simulink model "SwarmSMC1"  (R2022a)
settings: Solver=FixedStepAuto  StartTime=0.0  StopTime=50  FixedStep=0.001  RelTol=1e-3
libraries: slpidlib x26
(part 1 of 3)
settings Model: SimulationMode=rapid-accelerator  Creator=贺嘉辣  LastModifiedBy=YYL
settings SolverCC: AlgebraicLoopSolver=TrustRegion
settings DebuggingCC: UnconnectedInputMsg=warning  UnconnectedOutputMsg=warning  UnconnectedLineMsg=warning  SFMachineParentedDataDiag=warning
settings RTWCC: DLArmComputeVersion=19.05

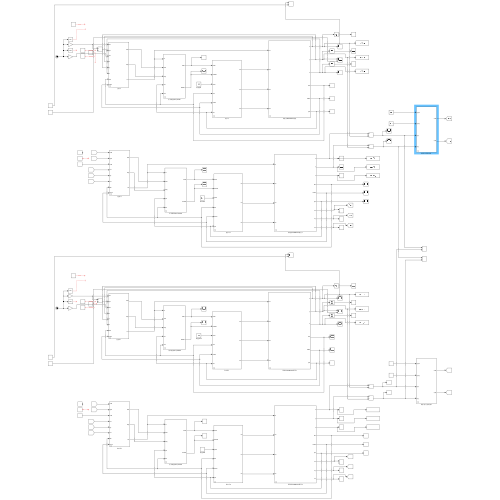
[thumbnail: Simulink's stored preview of the top-level diagram]
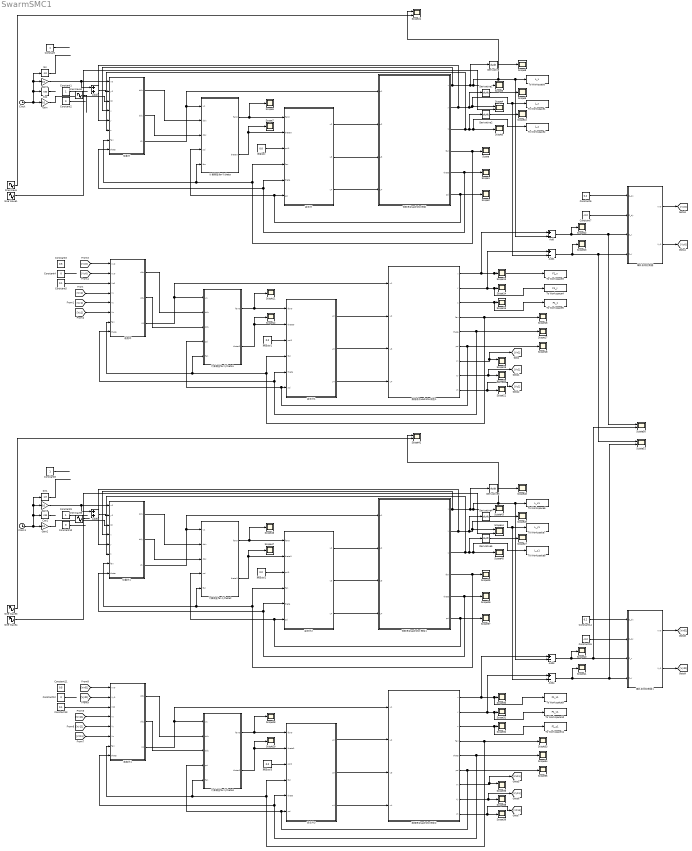
== system SwarmSMC1 ==
  Add{,1,3..4} (4 alike) : Sum  Inputs=+-
  Add2 : Sum
  Add5 : Sum
  Clock : Clock
  Clock1 : Clock
  Constant{,1,8..9} (4 alike) : Constant
  Constant{2,4,10,12} (4 alike) : Constant  Value=0
  Constant11 : Constant  Value=0.5
  Constant13 : Constant  Value=0.1
  Constant14 : Constant  Value=0.2
  Constant15 : Constant  Value=-0.2
  Constant3 : Constant  Value=0.5
  Constant5 : Constant  Value=0.1
  Constant6 : Constant  Value=0.2
  Constant7 : Constant  Value=-0.2
  Cos : Trigonometry  Operator=cos
  Cos1 : Trigonometry  Operator=cos
  Derivative{,1..5} (6 alike) : Derivative
  Gain{,1..3} (4 alike) : Gain  Gain=0.1
  Scope{,1..3,5..18,20..23,25..35,37..41,43,45..49} (44 alike) : Scope
  Scope{4,19,24,36,42,44,50..51} (8 alike) : Scope  NumInputPorts=2
  Sin : Trigonometry
  Sin1 : Trigonometry
  Sine Wave : Sin  Frequency=0.2  SampleTime=0
  Sine Wave1 : Sin  Frequency=0.2  Phase=pi/2  SampleTime=0
  Sine Wave2 : Sin  Amplitude=2.5  Frequency=0.04  SampleTime=0
  Sine Wave3 : Sin  Frequency=0.2  SampleTime=0
  Sine Wave4 : Sin  Frequency=0.2  Phase=pi/2  SampleTime=0
  Sine Wave5 : Sin  Amplitude=2.5  Frequency=0.04  SampleTime=0
  To Workspace : ToWorkspace  VariableName=L_x  SaveFormat=Timeseries  SampleTime=-1
  To Workspace1 : ToWorkspace  VariableName=L_y  SaveFormat=Timeseries  SampleTime=-1
  To Workspace10 : ToWorkspace  VariableName=F1_y1  SaveFormat=Timeseries  SampleTime=-1
  To Workspace11 : ToWorkspace  VariableName=F1_z1  SaveFormat=Timeseries  SampleTime=-1
  To Workspace2 : ToWorkspace  VariableName=L_z  SaveFormat=Timeseries  SampleTime=-1
  To Workspace3 : ToWorkspace  VariableName=F1_x  SaveFormat=Timeseries  SampleTime=-1
  To Workspace4 : ToWorkspace  VariableName=F1_y  SaveFormat=Timeseries  SampleTime=-1
  To Workspace5 : ToWorkspace  VariableName=F1_z  SaveFormat=Timeseries  SampleTime=-1
  To Workspace6 : ToWorkspace  VariableName=L_x1  SaveFormat=Timeseries  SampleTime=-1
  To Workspace7 : ToWorkspace  VariableName=L_y1  SaveFormat=Timeseries  SampleTime=-1
  To Workspace8 : ToWorkspace  VariableName=L_z1  SaveFormat=Timeseries  SampleTime=-1
  To Workspace9 : ToWorkspace  VariableName=F1_x1  SaveFormat=Timeseries  SampleTime=-1
  位置环 : Subsystem  mask{m=0.65, g=9.8}
      mask prompts: m "无人机质量"; g "重力加速度"
  位置环1 : Subsystem  mask{m=0.65, g=9.8}
      mask prompts: m "无人机质量"; g "重力加速度"
  姿态环 : Subsystem  mask{Ixx=7.5e-3, Iyy=7.5e-3, Izz=1.3e-2}
      mask prompts: Ixx "无人机绕X轴转动惯量"; Iyy "无人机绕Y轴转动惯量"; Izz "无人机绕Z轴转动惯量"
  姿态环1 : Subsystem  mask{Ixx=7.5e-3, Iyy=7.5e-3, Izz=1.3e-2}
      mask prompts: Ixx "无人机绕X轴转动惯量"; Iyy "无人机绕Y轴转动惯量"; Izz "无人机绕Z轴转动惯量"
  姿态环2 : Subsystem  mask{Ixx=7.5e-3, Iyy=7.5e-3, Izz=1.3e-2}
      mask prompts: Ixx "无人机绕X轴转动惯量"; Iyy "无人机绕Y轴转动惯量"; Izz "无人机绕Z轴转动惯量"
  姿态环3 : Subsystem  mask{Ixx=7.5e-3, Iyy=7.5e-3, Izz=1.3e-2}
      mask prompts: Ixx "无人机绕X轴转动惯量"; Iyy "无人机绕Y轴转动惯量"; Izz "无人机绕Z轴转动惯量"
  期望psi{,1..3} (4 alike) : Constant  Value=0.0
  编队协同控制器 : Subsystem  mask{m=0.65, g=9.8}
      mask prompts: m "无人机质量"; g "重力加速度"
  编队协同控制器1 : Subsystem  mask{m=0.65, g=9.8}
      mask prompts: m "无人机质量"; g "重力加速度"
  计算期望fan与theta : Subsystem  mask{m=0.65}
      mask prompts: m "无人机质量"
  计算期望fan与theta1 : Subsystem  mask{m=0.65}
      mask prompts: m "无人机质量"
  计算期望fan与theta2 : Subsystem  mask{m=0.65}
      mask prompts: m "无人机质量"
  计算期望fan与theta3 : Subsystem  mask{m=0.65}
      mask prompts: m "无人机质量"
  跟随者Quadrotor模型1 : Subsystem  mask{m=0.65, g=9.8, Ixx=7.5e-3, Iyy=7.5e-3, Izz=1.3e-2, L=0.23, rho=3.1e-5, gama=7.5e-7}
      mask prompts: m "无人机质量"; g "重力加速度"; Ixx "四旋翼绕X轴转动惯量"; Iyy "四旋翼绕Y轴转动惯量"; Izz "四旋翼绕Z轴转动惯量"; L "四旋翼臂长"; rho "四旋翼升力系数"; gama "空气阻力系数"
  跟随者Quadrotor模型2 : Subsystem  mask{m=0.65, g=9.8, Ixx=7.5e-3, Iyy=7.5e-3, Izz=1.3e-2, L=0.23, rho=3.1e-5, gama=7.5e-7}
      mask prompts: m "无人机质量"; g "重力加速度"; Ixx "四旋翼绕X轴转动惯量"; Iyy "四旋翼绕Y轴转动惯量"; Izz "四旋翼绕Z轴转动惯量"; L "四旋翼臂长"; rho "四旋翼升力系数"; gama "空气阻力系数"
  速度环 : Subsystem  mask{m=0.65, g=9.8}
      mask prompts: m "无人机质量"; g "重力加速度"
  速度环1 : Subsystem  mask{m=0.65, g=9.8}
      mask prompts: m "无人机质量"; g "重力加速度"
  领航者Quadrotor模型 : Subsystem  mask{m=0.65, g=9.8, Ixx=7.5e-3, Iyy=7.5e-3, Izz=1.3e-2, L=0.23, rho=3.1e-5, gama=7.5e-7}
      mask prompts: m "无人机质量"; g "重力加速度"; Ixx "四旋翼绕X轴转动惯量"; Iyy "四旋翼绕Y轴转动惯量"; Izz "四旋翼绕Z轴转动惯量"; L "四旋翼臂长"; rho "四旋翼升力系数"; gama "空气阻力系数"
  领航者Quadrotor模型1 : Subsystem  mask{m=0.65, g=9.8, Ixx=7.5e-3, Iyy=7.5e-3, Izz=1.3e-2, L=0.23, rho=3.1e-5, gama=7.5e-7}
      mask prompts: m "无人机质量"; g "重力加速度"; Ixx "四旋翼绕X轴转动惯量"; Iyy "四旋翼绕Y轴转动惯量"; Izz "四旋翼绕Z轴转动惯量"; L "四旋翼臂长"; rho "四旋翼升力系数"; gama "空气阻力系数"
  wires:
  姿态环/3(u4) -> 领航者Quadrotor模型/4(u4)
  姿态环/2(u3) -> 领航者Quadrotor模型/3(u3)
  姿态环/1(u2) -> 领航者Quadrotor模型/2(u2)
  领航者Quadrotor模型/5(theta) -> Scope1/1, 位置环/8(theta), 姿态环/5(theta)
  领航者Quadrotor模型/6(psi) -> Scope2/1, 计算期望fan与theta/4(psi), 姿态环/6(psi)
  领航者Quadrotor模型/4(fan) -> Scope/1, 姿态环/4(fan), 位置环/7(fan), 计算期望fan与theta/5(fan)
  领航者Quadrotor模型/1(x) -> 位置环/4(x), Derivative/1, Scope24/1, Add/2, To Workspace/1, Scope3/1
  领航者Quadrotor模型/2(y) -> 位置环/5(y), Derivative1/1, Scope4/1, Add1/2, To Workspace1/1
  领航者Quadrotor模型/3(z) -> 位置环/6(z), Derivative2/1, To Workspace2/1, Scope5/1
  期望psi/1 -> 姿态环/3(psi0)
  计算期望fan与theta/2(theta0) -> Scope7/1, 姿态环/2(theta0)
  计算期望fan与theta/1(fan0) -> 姿态环/1(fan0), Scope6/1
  位置环/1(ddx) -> 计算期望fan与theta/2(ddx)
  位置环/2(ddy) -> 计算期望fan与theta/3(ddy)
  位置环/3(U1) -> 领航者Quadrotor模型/1(u1), 计算期望fan与theta/1(u1)
  Clock/1 -> Gain/1, Gain1/1, Sin/1, Cos/1
  Constant/1 -> ?
  Constant1/1 -> ?
  Constant2/1 -> ?
  Derivative/1 -> Scope8/1
  Derivative1/1 -> Scope9/1
  Derivative2/1 -> Scope10/1
  [Vx1] -> 速度环/4(Vx)
  [Vy1] -> 速度环/5(Vy)
  [Vz1] -> 速度环/6(Vz)
  Constant5/1 -> 速度环/3(Vz0)
  Constant4/1 -> ?
  速度环/3(U1) -> 跟随者Quadrotor模型1/1(u1), 计算期望fan与theta1/1(u1)
  计算期望fan与theta1/1(fan0) -> Scope11/1, 姿态环1/1(fan0)
  计算期望fan与theta1/2(theta0) -> Scope12/1, 姿态环1/2(theta0)
  期望psi1/1 -> 姿态环1/3(psi0)
  姿态环1/1(u2) -> 跟随者Quadrotor模型1/2(u2)
  姿态环1/2(u3) -> 跟随者Quadrotor模型1/3(u3)
  姿态环1/3(u4) -> 跟随者Quadrotor模型1/4(u4)
  跟随者Quadrotor模型1/1(x) -> To Workspace3/1, Scope13/1, Add/1
  跟随者Quadrotor模型1/2(y) -> Add1/1, To Workspace4/1, Scope14/1
  跟随者Quadrotor模型1/3(z) -> To Workspace5/1, Scope15/1
  跟随者Quadrotor模型1/5(theta) -> 速度环/8(theta), 姿态环1/5(theta), Scope17/1
  跟随者Quadrotor模型1/6(psi) -> 姿态环1/6(psi), 计算期望fan与theta1/4(psi), Scope18/1
  跟随者Quadrotor模型1/7(Vx) -> Scope19/1, [Vx1]
  跟随者Quadrotor模型1/8(Vy) -> [Vy1], Scope20/1
  跟随者Quadrotor模型1/9(Vz) -> [Vz1], Scope21/1
  跟随者Quadrotor模型1/4(fan) -> Scope16/1, 姿态环1/4(fan), 计算期望fan与theta1/5(fan), 速度环/7(fan)
  Constant6/1 -> 编队协同控制器/1(S_dx)
  Constant7/1 -> 编队协同控制器/2(S_dy)
  Add1/1 -> Scope23/1, Scope51/1, 编队协同控制器/4(S_y)
  编队协同控制器/1(Vx0) -> [Vx0]
  编队协同控制器/2(Vy0) -> [Vy0]
  Sine Wave/1 -> Scope24/2
  Sin/1 -> ?
  Cos/1 -> ?
  Gain/1 -> 位置环/3(z0)
  速度环/1(ddx) -> 计算期望fan与theta1/2(ddx)
  速度环/2(ddy) -> 计算期望fan与theta1/3(ddy)
  [Vx0] -> 速度环/1(Vx0)
  [Vy0] -> 速度环/2(Vy0)
  Sine Wave1/1 -> Scope4/2
  Gain1/1 -> Add2/1, 位置环/1(x0)
  Add2/1 -> 位置环/2(y0)
  Sine Wave2/1 -> ?
  Constant8/1 -> ?
  Constant9/1 -> ?
  Constant10/1 -> ?
  Sin1/1 -> ?
  Constant12/1 -> ?
  Cos1/1 -> ?
  跟随者Quadrotor模型2/8(Vy) -> [Vy11], Scope38/1
  姿态环3/2(u3) -> 跟随者Quadrotor模型2/3(u3)
  Sine Wave5/1 -> ?
  Add5/1 -> 位置环1/2(y0)
  [Vx01] -> 速度环1/1(Vx0)
  跟随者Quadrotor模型2/2(y) -> Add4/1, To Workspace10/1, Scope31/1
  跟随者Quadrotor模型2/3(z) -> To Workspace11/1, Scope32/1
  领航者Quadrotor模型1/1(x) -> 位置环1/4(x), Derivative3/1, Scope42/1, Add3/2, To Workspace6/1, Scope43/1
  Gain3/1 -> Add5/1, 位置环1/1(x0)
  [Vy01] -> 速度环1/2(Vy0)
  [Vz11] -> 速度环1/6(Vz)
  跟随者Quadrotor模型2/5(theta) -> 速度环1/8(theta), 姿态环3/5(theta), Scope34/1
  位置环1/3(U1) -> 领航者Quadrotor模型1/1(u1), 计算期望fan与theta2/1(u1)
  [Vx11] -> 速度环1/4(Vx)
  编队协同控制器1/1(Vx0) -> [Vx01]
  Gain2/1 -> 位置环1/3(z0)
  Sine Wave4/1 -> Scope44/2
  计算期望fan与theta3/2(theta0) -> Scope29/1, 姿态环3/2(theta0)
  编队协同控制器1/2(Vy0) -> [Vy01]
  Add4/1 -> Scope41/1, Scope51/2, 编队协同控制器1/4(S_y)
  Constant15/1 -> 编队协同控制器1/2(S_dy)
  [Vy11] -> 速度环1/5(Vy)
  速度环1/1(ddx) -> 计算期望fan与theta3/2(ddx)
  Derivative3/1 -> Scope48/1
  Sine Wave3/1 -> Scope42/2
  跟随者Quadrotor模型2/6(psi) -> 姿态环3/6(psi), 计算期望fan与theta3/4(psi), Scope35/1
  跟随者Quadrotor模型2/1(x) -> To Workspace9/1, Scope30/1, Add3/1
  Constant14/1 -> 编队协同控制器1/1(S_dx)
  速度环1/3(U1) -> 跟随者Quadrotor模型2/1(u1), 计算期望fan与theta3/1(u1)
  姿态环3/1(u2) -> 跟随者Quadrotor模型2/2(u2)
  跟随者Quadrotor模型2/9(Vz) -> [Vz11], Scope39/1
  姿态环2/3(u4) -> 领航者Quadrotor模型1/4(u4)
  期望psi3/1 -> 姿态环3/3(psi0)
  计算期望fan与theta2/2(theta0) -> Scope47/1, 姿态环2/2(theta0)
  Constant13/1 -> 速度环1/3(Vz0)
  期望psi2/1 -> 姿态环2/3(psi0)
  姿态环2/1(u2) -> 领航者Quadrotor模型1/2(u2)
  计算期望fan与theta3/1(fan0) -> Scope28/1, 姿态环3/1(fan0)
  跟随者Quadrotor模型2/7(Vx) -> Scope36/1, [Vx11]
  Clock1/1 -> Gain2/1, Gain3/1, Sin1/1, Cos1/1
  位置环1/2(ddy) -> 计算期望fan与theta2/3(ddy)
  Derivative4/1 -> Scope49/1
  领航者Quadrotor模型1/3(z) -> 位置环1/6(z), Derivative5/1, To Workspace8/1, Scope45/1
  位置环1/1(ddx) -> 计算期望fan与theta2/2(ddx)
  姿态环3/3(u4) -> 跟随者Quadrotor模型2/4(u4)
  计算期望fan与theta2/1(fan0) -> 姿态环2/1(fan0), Scope46/1
  领航者Quadrotor模型1/4(fan) -> Scope25/1, 姿态环2/4(fan), 位置环1/7(fan), 计算期望fan与theta2/5(fan)
  速度环1/2(ddy) -> 计算期望fan与theta3/3(ddy)
  Derivative5/1 -> Scope27/1
  跟随者Quadrotor模型2/4(fan) -> Scope33/1, 姿态环3/4(fan), 计算期望fan与theta3/5(fan), 速度环1/7(fan)
  领航者Quadrotor模型1/2(y) -> 位置环1/5(y), Derivative4/1, Scope44/1, Add4/2, To Workspace7/1
  姿态环2/2(u3) -> 领航者Quadrotor模型1/3(u3)
  领航者Quadrotor模型1/5(theta) -> Scope26/1, 位置环1/8(theta), 姿态环2/5(theta)
  领航者Quadrotor模型1/6(psi) -> Scope37/1, 计算期望fan与theta2/4(psi), 姿态环2/6(psi)
  Add3/1 -> Scope40/1, Scope50/2, 编队协同控制器1/3(S_x)
  Add/1 -> Scope22/1, Scope50/1, 编队协同控制器/3(S_x)

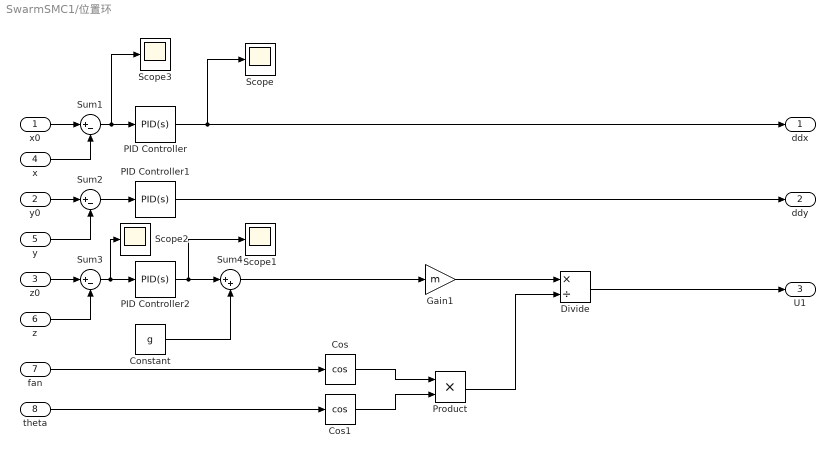
== system SwarmSMC1/位置环 ==
  x0 : Inport
  y0 : Inport  Port=2
  z0 : Inport  Port=3
  x : Inport  Port=4
  y : Inport  Port=5
  z : Inport  Port=6
  fan : Inport  Port=7
  theta : Inport  Port=8
  Constant : Constant  Value=g
  Cos : Trigonometry  Operator=cos
  Cos1 : Trigonometry  Operator=cos
  Divide : Product  Inputs=*/
  Gain1 : Gain  Gain=m
  PID Controller : slpidlib/PID Controller  Controller=PID  Form=Parallel  TimeDomain=Continuous-time  UseExternalTs=off  SampleTime=-1  IntegratorMethod=Forward Euler  FilterMethod=Forward Euler  ControllerParametersSource=internal  P=5  I=0  UseKiTs=off  D=15  N=1581.76882497108  UseFilter=on  TunerSelectOption=Transfer Function Based (PID Tuner App)  InitialConditionSource=internal  InitialConditionForIntegrator=0  InitialConditionForFilter=0  DifferentiatorICPrevScaledInput=0  ExternalReset=none  TrackingMode=off  Kt=1  LimitOutput=off  SatLimitsSource=internal  UpperSaturationLimit=inf  LowerSaturationLimit=-inf  LinearizeAsGain=on  AntiWindupMode=none  Kb=1  POutMin=[]  POutMax=[]  IOutMin=[]  IOutMax=[]  DOutMin=[]  DOutMax=[]  NOutMin=[]  NOutMax=[]  SumOutMin=[]  SumOutMax=[]  SaturationOutMin=[]  SaturationOutMax=[]  PParamMin=[]  PParamMax=[]  IParamMin=[]  IParamMax=[]  DParamMin=[]  DParamMax=[]  NParamMin=[]  NParamMax=[]  KbParamMin=[]  KbParamMax=[]  KtParamMin=[]  KtParamMax=[]  KbOutMin=[]  KbOutMax=[]  KtOutMin=[]  KtOutMax=[]  IntegratorOutMin=[]  IntegratorOutMax=[]  FilterOutMin=[]  FilterOutMax=[]  SumI1OutMin=[]  SumI1OutMax=[]  SumI2OutMin=[]  SumI2OutMax=[]  SumI3OutMin=[]  SumI3OutMax=[]  SumI4OutMin=[]  SumI4OutMax=[]  SumDOutMin=[]  SumDOutMax=[]  DifferentiatorOutMin=[]  DifferentiatorOutMax=[]  FilterDiffOutCoefMin=[]  FilterDiffOutCoefMax=[]  ReciprocalOutMin=[]  ReciprocalOutMax=[]  SumDenOutMin=[]  SumDenOutMax=[]  SumNumOutMin=[]  SumNumOutMax=[]  DivideOutMin=[]  DivideOutMax=[]  UdiffTsProdOutMin=[]  UdiffTsProdOutMax=[]  NTsProdOutMin=[]  NTsProdOutMax=[]  UintegralTsProdOutMin=[]  UintegralTsProdOutMax=[]  UngainTsProdOutMin=[]  UngainTsProdOutMax=[]  IntegratorContinuousStateAttributes=''  IntegratorStateMustResolveToSignalObject=off  IntegratorRTWStateStorageClass=Auto  FilterContinuousStateAttributes=''  FilterStateMustResolveToSignalObject=off  FilterRTWStateStorageClass=Auto  ParallelPVariant=InternalParameters  IdealPVariant=Disabled  IVariant=InternalParameters  DVariant=InternalParameters  IntegratorVariant=Continuous  SatVariant=Disabled  AWVariant=Passthrough  PCopyVariant=Disabled  TRVariant=Disabled  FdbkBlocksVariant=Forward  IdealPFdbkVariant=Disabled  SatFdbkVariant=Disabled  DerivativeFilterVariant=ContFilter  NVariant=InternalParameters  NCopyVariant=Disabled  FilterICVariant=InternalICsFilter  IntegratorICVariant=InternalICs  ExternalResetVariant=Disabled  TRSumVariant=Passthrough  SumFdbkVariant=Disabled  SumVariant=Sum_PID  TsampFilterVariant=InternalTs  TsampNgainVariant=Passthrough  TsampIntegralVariant=Passthrough  ExternalSaturationOutDataTypeStr=Inherit: Same as second input  aMode=0
  PID Controller1 : slpidlib/PID Controller  Controller=PID  Form=Parallel  TimeDomain=Continuous-time  UseExternalTs=off  SampleTime=-1  IntegratorMethod=Forward Euler  FilterMethod=Forward Euler  ControllerParametersSource=internal  P=5  I=0  UseKiTs=off  D=15  N=100  UseFilter=on  TunerSelectOption=Transfer Function Based (PID Tuner App)  InitialConditionSource=internal  InitialConditionForIntegrator=0  InitialConditionForFilter=0  DifferentiatorICPrevScaledInput=0  ExternalReset=none  TrackingMode=off  Kt=1  LimitOutput=off  SatLimitsSource=internal  UpperSaturationLimit=inf  LowerSaturationLimit=-inf  LinearizeAsGain=on  AntiWindupMode=none  Kb=1  POutMin=[]  POutMax=[]  IOutMin=[]  IOutMax=[]  DOutMin=[]  DOutMax=[]  NOutMin=[]  NOutMax=[]  SumOutMin=[]  SumOutMax=[]  SaturationOutMin=[]  SaturationOutMax=[]  PParamMin=[]  PParamMax=[]  IParamMin=[]  IParamMax=[]  DParamMin=[]  DParamMax=[]  NParamMin=[]  NParamMax=[]  KbParamMin=[]  KbParamMax=[]  KtParamMin=[]  KtParamMax=[]  KbOutMin=[]  KbOutMax=[]  KtOutMin=[]  KtOutMax=[]  IntegratorOutMin=[]  IntegratorOutMax=[]  FilterOutMin=[]  FilterOutMax=[]  SumI1OutMin=[]  SumI1OutMax=[]  SumI2OutMin=[]  SumI2OutMax=[]  SumI3OutMin=[]  SumI3OutMax=[]  SumI4OutMin=[]  SumI4OutMax=[]  SumDOutMin=[]  SumDOutMax=[]  DifferentiatorOutMin=[]  DifferentiatorOutMax=[]  FilterDiffOutCoefMin=[]  FilterDiffOutCoefMax=[]  ReciprocalOutMin=[]  ReciprocalOutMax=[]  SumDenOutMin=[]  SumDenOutMax=[]  SumNumOutMin=[]  SumNumOutMax=[]  DivideOutMin=[]  DivideOutMax=[]  UdiffTsProdOutMin=[]  UdiffTsProdOutMax=[]  NTsProdOutMin=[]  NTsProdOutMax=[]  UintegralTsProdOutMin=[]  UintegralTsProdOutMax=[]  UngainTsProdOutMin=[]  UngainTsProdOutMax=[]  IntegratorContinuousStateAttributes=''  IntegratorStateMustResolveToSignalObject=off  IntegratorRTWStateStorageClass=Auto  FilterContinuousStateAttributes=''  FilterStateMustResolveToSignalObject=off  FilterRTWStateStorageClass=Auto  ParallelPVariant=InternalParameters  IdealPVariant=Disabled  IVariant=InternalParameters  DVariant=InternalParameters  IntegratorVariant=Continuous  SatVariant=Disabled  AWVariant=Passthrough  PCopyVariant=Disabled  TRVariant=Disabled  FdbkBlocksVariant=Forward  IdealPFdbkVariant=Disabled  SatFdbkVariant=Disabled  DerivativeFilterVariant=ContFilter  NVariant=InternalParameters  NCopyVariant=Disabled  FilterICVariant=InternalICsFilter  IntegratorICVariant=InternalICs  ExternalResetVariant=Disabled  TRSumVariant=Passthrough  SumFdbkVariant=Disabled  SumVariant=Sum_PID  TsampFilterVariant=InternalTs  TsampNgainVariant=Passthrough  TsampIntegralVariant=Passthrough  ExternalSaturationOutDataTypeStr=Inherit: Same as second input  aMode=0
  PID Controller2 : slpidlib/PID Controller  Controller=PID  Form=Parallel  TimeDomain=Continuous-time  UseExternalTs=off  SampleTime=-1  IntegratorMethod=Forward Euler  FilterMethod=Forward Euler  ControllerParametersSource=internal  P=5  I=1.2  UseKiTs=off  D=4  N=100  UseFilter=on  TunerSelectOption=Transfer Function Based (PID Tuner App)  InitialConditionSource=internal  InitialConditionForIntegrator=0  InitialConditionForFilter=0  DifferentiatorICPrevScaledInput=0  ExternalReset=none  TrackingMode=off  Kt=1  LimitOutput=off  SatLimitsSource=internal  UpperSaturationLimit=inf  LowerSaturationLimit=-inf  LinearizeAsGain=on  AntiWindupMode=none  Kb=1  POutMin=[]  POutMax=[]  IOutMin=[]  IOutMax=[]  DOutMin=[]  DOutMax=[]  NOutMin=[]  NOutMax=[]  SumOutMin=[]  SumOutMax=[]  SaturationOutMin=[]  SaturationOutMax=[]  PParamMin=[]  PParamMax=[]  IParamMin=[]  IParamMax=[]  DParamMin=[]  DParamMax=[]  NParamMin=[]  NParamMax=[]  KbParamMin=[]  KbParamMax=[]  KtParamMin=[]  KtParamMax=[]  KbOutMin=[]  KbOutMax=[]  KtOutMin=[]  KtOutMax=[]  IntegratorOutMin=[]  IntegratorOutMax=[]  FilterOutMin=[]  FilterOutMax=[]  SumI1OutMin=[]  SumI1OutMax=[]  SumI2OutMin=[]  SumI2OutMax=[]  SumI3OutMin=[]  SumI3OutMax=[]  SumI4OutMin=[]  SumI4OutMax=[]  SumDOutMin=[]  SumDOutMax=[]  DifferentiatorOutMin=[]  DifferentiatorOutMax=[]  FilterDiffOutCoefMin=[]  FilterDiffOutCoefMax=[]  ReciprocalOutMin=[]  ReciprocalOutMax=[]  SumDenOutMin=[]  SumDenOutMax=[]  SumNumOutMin=[]  SumNumOutMax=[]  DivideOutMin=[]  DivideOutMax=[]  UdiffTsProdOutMin=[]  UdiffTsProdOutMax=[]  NTsProdOutMin=[]  NTsProdOutMax=[]  UintegralTsProdOutMin=[]  UintegralTsProdOutMax=[]  UngainTsProdOutMin=[]  UngainTsProdOutMax=[]  IntegratorContinuousStateAttributes=''  IntegratorStateMustResolveToSignalObject=off  IntegratorRTWStateStorageClass=Auto  FilterContinuousStateAttributes=''  FilterStateMustResolveToSignalObject=off  FilterRTWStateStorageClass=Auto  ParallelPVariant=InternalParameters  IdealPVariant=Disabled  IVariant=InternalParameters  DVariant=InternalParameters  IntegratorVariant=Continuous  SatVariant=Disabled  AWVariant=Passthrough  PCopyVariant=Disabled  TRVariant=Disabled  FdbkBlocksVariant=Forward  IdealPFdbkVariant=Disabled  SatFdbkVariant=Disabled  DerivativeFilterVariant=ContFilter  NVariant=InternalParameters  NCopyVariant=Disabled  FilterICVariant=InternalICsFilter  IntegratorICVariant=InternalICs  ExternalResetVariant=Disabled  TRSumVariant=Passthrough  SumFdbkVariant=Disabled  SumVariant=Sum_PID  TsampFilterVariant=InternalTs  TsampNgainVariant=Passthrough  TsampIntegralVariant=Passthrough  ExternalSaturationOutDataTypeStr=Inherit: Same as second input  aMode=0
  Product : Product
  Scope{,1..3} (4 alike) : Scope
  Sum1 : Sum  Inputs=|+-
  Sum2 : Sum  Inputs=|+-
  Sum3 : Sum  Inputs=|+-
  Sum4 : Sum  Inputs=|++
  ddx : Outport
  ddy : Outport  Port=2
  U1 : Outport  Port=3
  wires:
  PID Controller/1 -> Scope/1, ddx/1
  PID Controller1/1 -> ddy/1
  x0/1 -> Sum1/1
  Sum1/1 -> Scope3/1, PID Controller/1
  x/1 -> Sum1/2
  y0/1 -> Sum2/1
  Sum2/1 -> PID Controller1/1
  y/1 -> Sum2/2
  z0/1 -> Sum3/1
  Sum3/1 -> Scope2/1, PID Controller2/1
  z/1 -> Sum3/2
  PID Controller2/1 -> Scope1/1, Sum4/1
  Constant/1 -> Sum4/2
  Gain1/1 -> Divide/1
  fan/1 -> Cos/1
  theta/1 -> Cos1/1
  Cos/1 -> Product/1
  Cos1/1 -> Product/2
  Product/1 -> Divide/2
  Divide/1 -> U1/1
  Sum4/1 -> Gain1/1

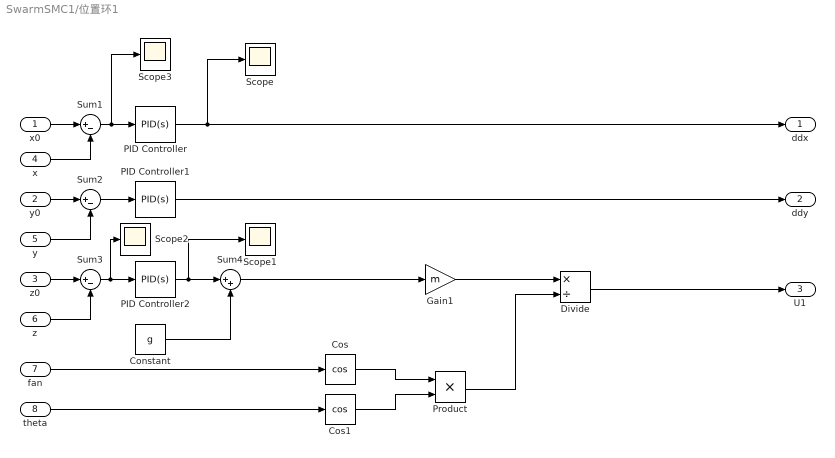
== system SwarmSMC1/位置环1 ==
  x0 : Inport
  y0 : Inport  Port=2
  z0 : Inport  Port=3
  x : Inport  Port=4
  y : Inport  Port=5
  z : Inport  Port=6
  fan : Inport  Port=7
  theta : Inport  Port=8
  Constant : Constant  Value=g
  Cos : Trigonometry  Operator=cos
  Cos1 : Trigonometry  Operator=cos
  Divide : Product  Inputs=*/
  Gain1 : Gain  Gain=m
  PID Controller : slpidlib/PID Controller  Controller=PID  Form=Parallel  TimeDomain=Continuous-time  UseExternalTs=off  SampleTime=-1  IntegratorMethod=Forward Euler  FilterMethod=Forward Euler  ControllerParametersSource=internal  P=5  I=0  UseKiTs=off  D=15  N=1581.76882497108  UseFilter=on  TunerSelectOption=Transfer Function Based (PID Tuner App)  InitialConditionSource=internal  InitialConditionForIntegrator=0  InitialConditionForFilter=0  DifferentiatorICPrevScaledInput=0  ExternalReset=none  TrackingMode=off  Kt=1  LimitOutput=off  SatLimitsSource=internal  UpperSaturationLimit=inf  LowerSaturationLimit=-inf  LinearizeAsGain=on  AntiWindupMode=none  Kb=1  POutMin=[]  POutMax=[]  IOutMin=[]  IOutMax=[]  DOutMin=[]  DOutMax=[]  NOutMin=[]  NOutMax=[]  SumOutMin=[]  SumOutMax=[]  SaturationOutMin=[]  SaturationOutMax=[]  PParamMin=[]  PParamMax=[]  IParamMin=[]  IParamMax=[]  DParamMin=[]  DParamMax=[]  NParamMin=[]  NParamMax=[]  KbParamMin=[]  KbParamMax=[]  KtParamMin=[]  KtParamMax=[]  KbOutMin=[]  KbOutMax=[]  KtOutMin=[]  KtOutMax=[]  IntegratorOutMin=[]  IntegratorOutMax=[]  FilterOutMin=[]  FilterOutMax=[]  SumI1OutMin=[]  SumI1OutMax=[]  SumI2OutMin=[]  SumI2OutMax=[]  SumI3OutMin=[]  SumI3OutMax=[]  SumI4OutMin=[]  SumI4OutMax=[]  SumDOutMin=[]  SumDOutMax=[]  DifferentiatorOutMin=[]  DifferentiatorOutMax=[]  FilterDiffOutCoefMin=[]  FilterDiffOutCoefMax=[]  ReciprocalOutMin=[]  ReciprocalOutMax=[]  SumDenOutMin=[]  SumDenOutMax=[]  SumNumOutMin=[]  SumNumOutMax=[]  DivideOutMin=[]  DivideOutMax=[]  UdiffTsProdOutMin=[]  UdiffTsProdOutMax=[]  NTsProdOutMin=[]  NTsProdOutMax=[]  UintegralTsProdOutMin=[]  UintegralTsProdOutMax=[]  UngainTsProdOutMin=[]  UngainTsProdOutMax=[]  IntegratorContinuousStateAttributes=''  IntegratorStateMustResolveToSignalObject=off  IntegratorRTWStateStorageClass=Auto  FilterContinuousStateAttributes=''  FilterStateMustResolveToSignalObject=off  FilterRTWStateStorageClass=Auto  ParallelPVariant=InternalParameters  IdealPVariant=Disabled  IVariant=InternalParameters  DVariant=InternalParameters  IntegratorVariant=Continuous  SatVariant=Disabled  AWVariant=Passthrough  PCopyVariant=Disabled  TRVariant=Disabled  FdbkBlocksVariant=Forward  IdealPFdbkVariant=Disabled  SatFdbkVariant=Disabled  DerivativeFilterVariant=ContFilter  NVariant=InternalParameters  NCopyVariant=Disabled  FilterICVariant=InternalICsFilter  IntegratorICVariant=InternalICs  ExternalResetVariant=Disabled  TRSumVariant=Passthrough  SumFdbkVariant=Disabled  SumVariant=Sum_PID  TsampFilterVariant=InternalTs  TsampNgainVariant=Passthrough  TsampIntegralVariant=Passthrough  ExternalSaturationOutDataTypeStr=Inherit: Same as second input  aMode=0
  PID Controller1 : slpidlib/PID Controller  Controller=PID  Form=Parallel  TimeDomain=Continuous-time  UseExternalTs=off  SampleTime=-1  IntegratorMethod=Forward Euler  FilterMethod=Forward Euler  ControllerParametersSource=internal  P=5  I=0  UseKiTs=off  D=15  N=100  UseFilter=on  TunerSelectOption=Transfer Function Based (PID Tuner App)  InitialConditionSource=internal  InitialConditionForIntegrator=0  InitialConditionForFilter=0  DifferentiatorICPrevScaledInput=0  ExternalReset=none  TrackingMode=off  Kt=1  LimitOutput=off  SatLimitsSource=internal  UpperSaturationLimit=inf  LowerSaturationLimit=-inf  LinearizeAsGain=on  AntiWindupMode=none  Kb=1  POutMin=[]  POutMax=[]  IOutMin=[]  IOutMax=[]  DOutMin=[]  DOutMax=[]  NOutMin=[]  NOutMax=[]  SumOutMin=[]  SumOutMax=[]  SaturationOutMin=[]  SaturationOutMax=[]  PParamMin=[]  PParamMax=[]  IParamMin=[]  IParamMax=[]  DParamMin=[]  DParamMax=[]  NParamMin=[]  NParamMax=[]  KbParamMin=[]  KbParamMax=[]  KtParamMin=[]  KtParamMax=[]  KbOutMin=[]  KbOutMax=[]  KtOutMin=[]  KtOutMax=[]  IntegratorOutMin=[]  IntegratorOutMax=[]  FilterOutMin=[]  FilterOutMax=[]  SumI1OutMin=[]  SumI1OutMax=[]  SumI2OutMin=[]  SumI2OutMax=[]  SumI3OutMin=[]  SumI3OutMax=[]  SumI4OutMin=[]  SumI4OutMax=[]  SumDOutMin=[]  SumDOutMax=[]  DifferentiatorOutMin=[]  DifferentiatorOutMax=[]  FilterDiffOutCoefMin=[]  FilterDiffOutCoefMax=[]  ReciprocalOutMin=[]  ReciprocalOutMax=[]  SumDenOutMin=[]  SumDenOutMax=[]  SumNumOutMin=[]  SumNumOutMax=[]  DivideOutMin=[]  DivideOutMax=[]  UdiffTsProdOutMin=[]  UdiffTsProdOutMax=[]  NTsProdOutMin=[]  NTsProdOutMax=[]  UintegralTsProdOutMin=[]  UintegralTsProdOutMax=[]  UngainTsProdOutMin=[]  UngainTsProdOutMax=[]  IntegratorContinuousStateAttributes=''  IntegratorStateMustResolveToSignalObject=off  IntegratorRTWStateStorageClass=Auto  FilterContinuousStateAttributes=''  FilterStateMustResolveToSignalObject=off  FilterRTWStateStorageClass=Auto  ParallelPVariant=InternalParameters  IdealPVariant=Disabled  IVariant=InternalParameters  DVariant=InternalParameters  IntegratorVariant=Continuous  SatVariant=Disabled  AWVariant=Passthrough  PCopyVariant=Disabled  TRVariant=Disabled  FdbkBlocksVariant=Forward  IdealPFdbkVariant=Disabled  SatFdbkVariant=Disabled  DerivativeFilterVariant=ContFilter  NVariant=InternalParameters  NCopyVariant=Disabled  FilterICVariant=InternalICsFilter  IntegratorICVariant=InternalICs  ExternalResetVariant=Disabled  TRSumVariant=Passthrough  SumFdbkVariant=Disabled  SumVariant=Sum_PID  TsampFilterVariant=InternalTs  TsampNgainVariant=Passthrough  TsampIntegralVariant=Passthrough  ExternalSaturationOutDataTypeStr=Inherit: Same as second input  aMode=0
  PID Controller2 : slpidlib/PID Controller  Controller=PID  Form=Parallel  TimeDomain=Continuous-time  UseExternalTs=off  SampleTime=-1  IntegratorMethod=Forward Euler  FilterMethod=Forward Euler  ControllerParametersSource=internal  P=5  I=1.2  UseKiTs=off  D=4  N=100  UseFilter=on  TunerSelectOption=Transfer Function Based (PID Tuner App)  InitialConditionSource=internal  InitialConditionForIntegrator=0  InitialConditionForFilter=0  DifferentiatorICPrevScaledInput=0  ExternalReset=none  TrackingMode=off  Kt=1  LimitOutput=off  SatLimitsSource=internal  UpperSaturationLimit=inf  LowerSaturationLimit=-inf  LinearizeAsGain=on  AntiWindupMode=none  Kb=1  POutMin=[]  POutMax=[]  IOutMin=[]  IOutMax=[]  DOutMin=[]  DOutMax=[]  NOutMin=[]  NOutMax=[]  SumOutMin=[]  SumOutMax=[]  SaturationOutMin=[]  SaturationOutMax=[]  PParamMin=[]  PParamMax=[]  IParamMin=[]  IParamMax=[]  DParamMin=[]  DParamMax=[]  NParamMin=[]  NParamMax=[]  KbParamMin=[]  KbParamMax=[]  KtParamMin=[]  KtParamMax=[]  KbOutMin=[]  KbOutMax=[]  KtOutMin=[]  KtOutMax=[]  IntegratorOutMin=[]  IntegratorOutMax=[]  FilterOutMin=[]  FilterOutMax=[]  SumI1OutMin=[]  SumI1OutMax=[]  SumI2OutMin=[]  SumI2OutMax=[]  SumI3OutMin=[]  SumI3OutMax=[]  SumI4OutMin=[]  SumI4OutMax=[]  SumDOutMin=[]  SumDOutMax=[]  DifferentiatorOutMin=[]  DifferentiatorOutMax=[]  FilterDiffOutCoefMin=[]  FilterDiffOutCoefMax=[]  ReciprocalOutMin=[]  ReciprocalOutMax=[]  SumDenOutMin=[]  SumDenOutMax=[]  SumNumOutMin=[]  SumNumOutMax=[]  DivideOutMin=[]  DivideOutMax=[]  UdiffTsProdOutMin=[]  UdiffTsProdOutMax=[]  NTsProdOutMin=[]  NTsProdOutMax=[]  UintegralTsProdOutMin=[]  UintegralTsProdOutMax=[]  UngainTsProdOutMin=[]  UngainTsProdOutMax=[]  IntegratorContinuousStateAttributes=''  IntegratorStateMustResolveToSignalObject=off  IntegratorRTWStateStorageClass=Auto  FilterContinuousStateAttributes=''  FilterStateMustResolveToSignalObject=off  FilterRTWStateStorageClass=Auto  ParallelPVariant=InternalParameters  IdealPVariant=Disabled  IVariant=InternalParameters  DVariant=InternalParameters  IntegratorVariant=Continuous  SatVariant=Disabled  AWVariant=Passthrough  PCopyVariant=Disabled  TRVariant=Disabled  FdbkBlocksVariant=Forward  IdealPFdbkVariant=Disabled  SatFdbkVariant=Disabled  DerivativeFilterVariant=ContFilter  NVariant=InternalParameters  NCopyVariant=Disabled  FilterICVariant=InternalICsFilter  IntegratorICVariant=InternalICs  ExternalResetVariant=Disabled  TRSumVariant=Passthrough  SumFdbkVariant=Disabled  SumVariant=Sum_PID  TsampFilterVariant=InternalTs  TsampNgainVariant=Passthrough  TsampIntegralVariant=Passthrough  ExternalSaturationOutDataTypeStr=Inherit: Same as second input  aMode=0
  Product : Product
  Scope{,1..3} (4 alike) : Scope
  Sum1 : Sum  Inputs=|+-
  Sum2 : Sum  Inputs=|+-
  Sum3 : Sum  Inputs=|+-
  Sum4 : Sum  Inputs=|++
  ddx : Outport
  ddy : Outport  Port=2
  U1 : Outport  Port=3
  wires:
  PID Controller/1 -> Scope/1, ddx/1
  PID Controller1/1 -> ddy/1
  x0/1 -> Sum1/1
  Sum1/1 -> Scope3/1, PID Controller/1
  x/1 -> Sum1/2
  y0/1 -> Sum2/1
  Sum2/1 -> PID Controller1/1
  y/1 -> Sum2/2
  z0/1 -> Sum3/1
  Sum3/1 -> Scope2/1, PID Controller2/1
  z/1 -> Sum3/2
  PID Controller2/1 -> Scope1/1, Sum4/1
  Constant/1 -> Sum4/2
  Gain1/1 -> Divide/1
  fan/1 -> Cos/1
  theta/1 -> Cos1/1
  Cos/1 -> Product/1
  Cos1/1 -> Product/2
  Product/1 -> Divide/2
  Divide/1 -> U1/1
  Sum4/1 -> Gain1/1

== system SwarmSMC1/姿态环 ==
  fan0 : Inport
  theta0 : Inport  Port=2
  psi0 : Inport  Port=3
  fan : Inport  Port=4
  theta : Inport  Port=5
  psi : Inport  Port=6
  Gain : Gain  Gain=Ixx
  Gain1 : Gain  Gain=Iyy
  Gain2 : Gain  Gain=Izz
  PID Controller : slpidlib/PID Controller  Controller=PID  Form=Parallel  TimeDomain=Continuous-time  UseExternalTs=off  SampleTime=-1  IntegratorMethod=Forward Euler  FilterMethod=Forward Euler  ControllerParametersSource=internal  P=74.27  I=69.54  UseKiTs=off  D=19.48  N=100  UseFilter=on  TunerSelectOption=Transfer Function Based (PID Tuner App)  InitialConditionSource=internal  InitialConditionForIntegrator=0  InitialConditionForFilter=0  DifferentiatorICPrevScaledInput=0  ExternalReset=none  TrackingMode=off  Kt=1  LimitOutput=off  SatLimitsSource=internal  UpperSaturationLimit=inf  LowerSaturationLimit=-inf  LinearizeAsGain=on  AntiWindupMode=none  Kb=1  POutMin=[]  POutMax=[]  IOutMin=[]  IOutMax=[]  DOutMin=[]  DOutMax=[]  NOutMin=[]  NOutMax=[]  SumOutMin=[]  SumOutMax=[]  SaturationOutMin=[]  SaturationOutMax=[]  PParamMin=[]  PParamMax=[]  IParamMin=[]  IParamMax=[]  DParamMin=[]  DParamMax=[]  NParamMin=[]  NParamMax=[]  KbParamMin=[]  KbParamMax=[]  KtParamMin=[]  KtParamMax=[]  KbOutMin=[]  KbOutMax=[]  KtOutMin=[]  KtOutMax=[]  IntegratorOutMin=[]  IntegratorOutMax=[]  FilterOutMin=[]  FilterOutMax=[]  SumI1OutMin=[]  SumI1OutMax=[]  SumI2OutMin=[]  SumI2OutMax=[]  SumI3OutMin=[]  SumI3OutMax=[]  SumI4OutMin=[]  SumI4OutMax=[]  SumDOutMin=[]  SumDOutMax=[]  DifferentiatorOutMin=[]  DifferentiatorOutMax=[]  FilterDiffOutCoefMin=[]  FilterDiffOutCoefMax=[]  ReciprocalOutMin=[]  ReciprocalOutMax=[]  SumDenOutMin=[]  SumDenOutMax=[]  SumNumOutMin=[]  SumNumOutMax=[]  DivideOutMin=[]  DivideOutMax=[]  UdiffTsProdOutMin=[]  UdiffTsProdOutMax=[]  NTsProdOutMin=[]  NTsProdOutMax=[]  UintegralTsProdOutMin=[]  UintegralTsProdOutMax=[]  UngainTsProdOutMin=[]  UngainTsProdOutMax=[]  IntegratorContinuousStateAttributes=''  IntegratorStateMustResolveToSignalObject=off  IntegratorRTWStateStorageClass=Auto  FilterContinuousStateAttributes=''  FilterStateMustResolveToSignalObject=off  FilterRTWStateStorageClass=Auto  ParallelPVariant=InternalParameters  IdealPVariant=Disabled  IVariant=InternalParameters  DVariant=InternalParameters  IntegratorVariant=Continuous  SatVariant=Disabled  AWVariant=Passthrough  PCopyVariant=Disabled  TRVariant=Disabled  FdbkBlocksVariant=Forward  IdealPFdbkVariant=Disabled  SatFdbkVariant=Disabled  DerivativeFilterVariant=ContFilter  NVariant=InternalParameters  NCopyVariant=Disabled  FilterICVariant=InternalICsFilter  IntegratorICVariant=InternalICs  ExternalResetVariant=Disabled  TRSumVariant=Passthrough  SumFdbkVariant=Disabled  SumVariant=Sum_PID  TsampFilterVariant=InternalTs  TsampNgainVariant=Passthrough  TsampIntegralVariant=Passthrough  ExternalSaturationOutDataTypeStr=Inherit: Same as second input  aMode=0
  PID Controller1 : slpidlib/PID Controller  Controller=PID  Form=Parallel  TimeDomain=Continuous-time  UseExternalTs=off  SampleTime=-1  IntegratorMethod=Forward Euler  FilterMethod=Forward Euler  ControllerParametersSource=internal  P=74.27  I=69.54  UseKiTs=off  D=19.48  N=100  UseFilter=on  TunerSelectOption=Transfer Function Based (PID Tuner App)  InitialConditionSource=internal  InitialConditionForIntegrator=0  InitialConditionForFilter=0  DifferentiatorICPrevScaledInput=0  ExternalReset=none  TrackingMode=off  Kt=1  LimitOutput=off  SatLimitsSource=internal  UpperSaturationLimit=inf  LowerSaturationLimit=-inf  LinearizeAsGain=on  AntiWindupMode=none  Kb=1  POutMin=[]  POutMax=[]  IOutMin=[]  IOutMax=[]  DOutMin=[]  DOutMax=[]  NOutMin=[]  NOutMax=[]  SumOutMin=[]  SumOutMax=[]  SaturationOutMin=[]  SaturationOutMax=[]  PParamMin=[]  PParamMax=[]  IParamMin=[]  IParamMax=[]  DParamMin=[]  DParamMax=[]  NParamMin=[]  NParamMax=[]  KbParamMin=[]  KbParamMax=[]  KtParamMin=[]  KtParamMax=[]  KbOutMin=[]  KbOutMax=[]  KtOutMin=[]  KtOutMax=[]  IntegratorOutMin=[]  IntegratorOutMax=[]  FilterOutMin=[]  FilterOutMax=[]  SumI1OutMin=[]  SumI1OutMax=[]  SumI2OutMin=[]  SumI2OutMax=[]  SumI3OutMin=[]  SumI3OutMax=[]  SumI4OutMin=[]  SumI4OutMax=[]  SumDOutMin=[]  SumDOutMax=[]  DifferentiatorOutMin=[]  DifferentiatorOutMax=[]  FilterDiffOutCoefMin=[]  FilterDiffOutCoefMax=[]  ReciprocalOutMin=[]  ReciprocalOutMax=[]  SumDenOutMin=[]  SumDenOutMax=[]  SumNumOutMin=[]  SumNumOutMax=[]  DivideOutMin=[]  DivideOutMax=[]  UdiffTsProdOutMin=[]  UdiffTsProdOutMax=[]  NTsProdOutMin=[]  NTsProdOutMax=[]  UintegralTsProdOutMin=[]  UintegralTsProdOutMax=[]  UngainTsProdOutMin=[]  UngainTsProdOutMax=[]  IntegratorContinuousStateAttributes=''  IntegratorStateMustResolveToSignalObject=off  IntegratorRTWStateStorageClass=Auto  FilterContinuousStateAttributes=''  FilterStateMustResolveToSignalObject=off  FilterRTWStateStorageClass=Auto  ParallelPVariant=InternalParameters  IdealPVariant=Disabled  IVariant=InternalParameters  DVariant=InternalParameters  IntegratorVariant=Continuous  SatVariant=Disabled  AWVariant=Passthrough  PCopyVariant=Disabled  TRVariant=Disabled  FdbkBlocksVariant=Forward  IdealPFdbkVariant=Disabled  SatFdbkVariant=Disabled  DerivativeFilterVariant=ContFilter  NVariant=InternalParameters  NCopyVariant=Disabled  FilterICVariant=InternalICsFilter  IntegratorICVariant=InternalICs  ExternalResetVariant=Disabled  TRSumVariant=Passthrough  SumFdbkVariant=Disabled  SumVariant=Sum_PID  TsampFilterVariant=InternalTs  TsampNgainVariant=Passthrough  TsampIntegralVariant=Passthrough  ExternalSaturationOutDataTypeStr=Inherit: Same as second input  aMode=0
  PID Controller2 : slpidlib/PID Controller  Controller=PID  Form=Parallel  TimeDomain=Continuous-time  UseExternalTs=off  SampleTime=-1  IntegratorMethod=Forward Euler  FilterMethod=Forward Euler  ControllerParametersSource=internal  P=160  I=30  UseKiTs=off  D=150  N=1000  UseFilter=on  TunerSelectOption=Transfer Function Based (PID Tuner App)  InitialConditionSource=internal  InitialConditionForIntegrator=0  InitialConditionForFilter=0  DifferentiatorICPrevScaledInput=0  ExternalReset=none  TrackingMode=off  Kt=1  LimitOutput=off  SatLimitsSource=internal  UpperSaturationLimit=inf  LowerSaturationLimit=-inf  LinearizeAsGain=on  AntiWindupMode=none  Kb=1  POutMin=[]  POutMax=[]  IOutMin=[]  IOutMax=[]  DOutMin=[]  DOutMax=[]  NOutMin=[]  NOutMax=[]  SumOutMin=[]  SumOutMax=[]  SaturationOutMin=[]  SaturationOutMax=[]  PParamMin=[]  PParamMax=[]  IParamMin=[]  IParamMax=[]  DParamMin=[]  DParamMax=[]  NParamMin=[]  NParamMax=[]  KbParamMin=[]  KbParamMax=[]  KtParamMin=[]  KtParamMax=[]  KbOutMin=[]  KbOutMax=[]  KtOutMin=[]  KtOutMax=[]  IntegratorOutMin=[]  IntegratorOutMax=[]  FilterOutMin=[]  FilterOutMax=[]  SumI1OutMin=[]  SumI1OutMax=[]  SumI2OutMin=[]  SumI2OutMax=[]  SumI3OutMin=[]  SumI3OutMax=[]  SumI4OutMin=[]  SumI4OutMax=[]  SumDOutMin=[]  SumDOutMax=[]  DifferentiatorOutMin=[]  DifferentiatorOutMax=[]  FilterDiffOutCoefMin=[]  FilterDiffOutCoefMax=[]  ReciprocalOutMin=[]  ReciprocalOutMax=[]  SumDenOutMin=[]  SumDenOutMax=[]  SumNumOutMin=[]  SumNumOutMax=[]  DivideOutMin=[]  DivideOutMax=[]  UdiffTsProdOutMin=[]  UdiffTsProdOutMax=[]  NTsProdOutMin=[]  NTsProdOutMax=[]  UintegralTsProdOutMin=[]  UintegralTsProdOutMax=[]  UngainTsProdOutMin=[]  UngainTsProdOutMax=[]  IntegratorContinuousStateAttributes=''  IntegratorStateMustResolveToSignalObject=off  IntegratorRTWStateStorageClass=Auto  FilterContinuousStateAttributes=''  FilterStateMustResolveToSignalObject=off  FilterRTWStateStorageClass=Auto  ParallelPVariant=InternalParameters  IdealPVariant=Disabled  IVariant=InternalParameters  DVariant=InternalParameters  IntegratorVariant=Continuous  SatVariant=Disabled  AWVariant=Passthrough  PCopyVariant=Disabled  TRVariant=Disabled  FdbkBlocksVariant=Forward  IdealPFdbkVariant=Disabled  SatFdbkVariant=Disabled  DerivativeFilterVariant=ContFilter  NVariant=InternalParameters  NCopyVariant=Disabled  FilterICVariant=InternalICsFilter  IntegratorICVariant=InternalICs  ExternalResetVariant=Disabled  TRSumVariant=Passthrough  SumFdbkVariant=Disabled  SumVariant=Sum_PID  TsampFilterVariant=InternalTs  TsampNgainVariant=Passthrough  TsampIntegralVariant=Passthrough  ExternalSaturationOutDataTypeStr=Inherit: Same as second input  aMode=0
  Sum : Sum  Inputs=|+-
  Sum1 : Sum  Inputs=|+-
  Sum2 : Sum  Inputs=|+-
  u2 : Outport
  u3 : Outport  Port=2
  u4 : Outport  Port=3
  wires:
  fan0/1 -> Sum/1
  fan/1 -> Sum/2
  theta0/1 -> Sum1/1
  theta/1 -> Sum1/2
  psi0/1 -> Sum2/1
  psi/1 -> Sum2/2
  Sum/1 -> PID Controller/1
  Sum1/1 -> PID Controller1/1
  Sum2/1 -> PID Controller2/1
  PID Controller/1 -> Gain/1
  Gain/1 -> u2/1
  PID Controller2/1 -> Gain2/1
  PID Controller1/1 -> Gain1/1
  Gain2/1 -> u4/1
  Gain1/1 -> u3/1

== system SwarmSMC1/姿态环1 ==
  fan0 : Inport
  theta0 : Inport  Port=2
  psi0 : Inport  Port=3
  fan : Inport  Port=4
  theta : Inport  Port=5
  psi : Inport  Port=6
  Gain : Gain  Gain=Ixx
  Gain1 : Gain  Gain=Iyy
  Gain2 : Gain  Gain=Izz
  PID Controller : slpidlib/PID Controller  Controller=PID  Form=Parallel  TimeDomain=Continuous-time  UseExternalTs=off  SampleTime=-1  IntegratorMethod=Forward Euler  FilterMethod=Forward Euler  ControllerParametersSource=internal  P=74.27  I=69.54  UseKiTs=off  D=19.48  N=100  UseFilter=on  TunerSelectOption=Transfer Function Based (PID Tuner App)  InitialConditionSource=internal  InitialConditionForIntegrator=0  InitialConditionForFilter=0  DifferentiatorICPrevScaledInput=0  ExternalReset=none  TrackingMode=off  Kt=1  LimitOutput=off  SatLimitsSource=internal  UpperSaturationLimit=inf  LowerSaturationLimit=-inf  LinearizeAsGain=on  AntiWindupMode=none  Kb=1  POutMin=[]  POutMax=[]  IOutMin=[]  IOutMax=[]  DOutMin=[]  DOutMax=[]  NOutMin=[]  NOutMax=[]  SumOutMin=[]  SumOutMax=[]  SaturationOutMin=[]  SaturationOutMax=[]  PParamMin=[]  PParamMax=[]  IParamMin=[]  IParamMax=[]  DParamMin=[]  DParamMax=[]  NParamMin=[]  NParamMax=[]  KbParamMin=[]  KbParamMax=[]  KtParamMin=[]  KtParamMax=[]  KbOutMin=[]  KbOutMax=[]  KtOutMin=[]  KtOutMax=[]  IntegratorOutMin=[]  IntegratorOutMax=[]  FilterOutMin=[]  FilterOutMax=[]  SumI1OutMin=[]  SumI1OutMax=[]  SumI2OutMin=[]  SumI2OutMax=[]  SumI3OutMin=[]  SumI3OutMax=[]  SumI4OutMin=[]  SumI4OutMax=[]  SumDOutMin=[]  SumDOutMax=[]  DifferentiatorOutMin=[]  DifferentiatorOutMax=[]  FilterDiffOutCoefMin=[]  FilterDiffOutCoefMax=[]  ReciprocalOutMin=[]  ReciprocalOutMax=[]  SumDenOutMin=[]  SumDenOutMax=[]  SumNumOutMin=[]  SumNumOutMax=[]  DivideOutMin=[]  DivideOutMax=[]  UdiffTsProdOutMin=[]  UdiffTsProdOutMax=[]  NTsProdOutMin=[]  NTsProdOutMax=[]  UintegralTsProdOutMin=[]  UintegralTsProdOutMax=[]  UngainTsProdOutMin=[]  UngainTsProdOutMax=[]  IntegratorContinuousStateAttributes=''  IntegratorStateMustResolveToSignalObject=off  IntegratorRTWStateStorageClass=Auto  FilterContinuousStateAttributes=''  FilterStateMustResolveToSignalObject=off  FilterRTWStateStorageClass=Auto  ParallelPVariant=InternalParameters  IdealPVariant=Disabled  IVariant=InternalParameters  DVariant=InternalParameters  IntegratorVariant=Continuous  SatVariant=Disabled  AWVariant=Passthrough  PCopyVariant=Disabled  TRVariant=Disabled  FdbkBlocksVariant=Forward  IdealPFdbkVariant=Disabled  SatFdbkVariant=Disabled  DerivativeFilterVariant=ContFilter  NVariant=InternalParameters  NCopyVariant=Disabled  FilterICVariant=InternalICsFilter  IntegratorICVariant=InternalICs  ExternalResetVariant=Disabled  TRSumVariant=Passthrough  SumFdbkVariant=Disabled  SumVariant=Sum_PID  TsampFilterVariant=InternalTs  TsampNgainVariant=Passthrough  TsampIntegralVariant=Passthrough  ExternalSaturationOutDataTypeStr=Inherit: Same as second input  aMode=0
  PID Controller1 : slpidlib/PID Controller  Controller=PID  Form=Parallel  TimeDomain=Continuous-time  UseExternalTs=off  SampleTime=-1  IntegratorMethod=Forward Euler  FilterMethod=Forward Euler  ControllerParametersSource=internal  P=74.27  I=69.54  UseKiTs=off  D=19.48  N=100  UseFilter=on  TunerSelectOption=Transfer Function Based (PID Tuner App)  InitialConditionSource=internal  InitialConditionForIntegrator=0  InitialConditionForFilter=0  DifferentiatorICPrevScaledInput=0  ExternalReset=none  TrackingMode=off  Kt=1  LimitOutput=off  SatLimitsSource=internal  UpperSaturationLimit=inf  LowerSaturationLimit=-inf  LinearizeAsGain=on  AntiWindupMode=none  Kb=1  POutMin=[]  POutMax=[]  IOutMin=[]  IOutMax=[]  DOutMin=[]  DOutMax=[]  NOutMin=[]  NOutMax=[]  SumOutMin=[]  SumOutMax=[]  SaturationOutMin=[]  SaturationOutMax=[]  PParamMin=[]  PParamMax=[]  IParamMin=[]  IParamMax=[]  DParamMin=[]  DParamMax=[]  NParamMin=[]  NParamMax=[]  KbParamMin=[]  KbParamMax=[]  KtParamMin=[]  KtParamMax=[]  KbOutMin=[]  KbOutMax=[]  KtOutMin=[]  KtOutMax=[]  IntegratorOutMin=[]  IntegratorOutMax=[]  FilterOutMin=[]  FilterOutMax=[]  SumI1OutMin=[]  SumI1OutMax=[]  SumI2OutMin=[]  SumI2OutMax=[]  SumI3OutMin=[]  SumI3OutMax=[]  SumI4OutMin=[]  SumI4OutMax=[]  SumDOutMin=[]  SumDOutMax=[]  DifferentiatorOutMin=[]  DifferentiatorOutMax=[]  FilterDiffOutCoefMin=[]  FilterDiffOutCoefMax=[]  ReciprocalOutMin=[]  ReciprocalOutMax=[]  SumDenOutMin=[]  SumDenOutMax=[]  SumNumOutMin=[]  SumNumOutMax=[]  DivideOutMin=[]  DivideOutMax=[]  UdiffTsProdOutMin=[]  UdiffTsProdOutMax=[]  NTsProdOutMin=[]  NTsProdOutMax=[]  UintegralTsProdOutMin=[]  UintegralTsProdOutMax=[]  UngainTsProdOutMin=[]  UngainTsProdOutMax=[]  IntegratorContinuousStateAttributes=''  IntegratorStateMustResolveToSignalObject=off  IntegratorRTWStateStorageClass=Auto  FilterContinuousStateAttributes=''  FilterStateMustResolveToSignalObject=off  FilterRTWStateStorageClass=Auto  ParallelPVariant=InternalParameters  IdealPVariant=Disabled  IVariant=InternalParameters  DVariant=InternalParameters  IntegratorVariant=Continuous  SatVariant=Disabled  AWVariant=Passthrough  PCopyVariant=Disabled  TRVariant=Disabled  FdbkBlocksVariant=Forward  IdealPFdbkVariant=Disabled  SatFdbkVariant=Disabled  DerivativeFilterVariant=ContFilter  NVariant=InternalParameters  NCopyVariant=Disabled  FilterICVariant=InternalICsFilter  IntegratorICVariant=InternalICs  ExternalResetVariant=Disabled  TRSumVariant=Passthrough  SumFdbkVariant=Disabled  SumVariant=Sum_PID  TsampFilterVariant=InternalTs  TsampNgainVariant=Passthrough  TsampIntegralVariant=Passthrough  ExternalSaturationOutDataTypeStr=Inherit: Same as second input  aMode=0
  PID Controller2 : slpidlib/PID Controller  Controller=PID  Form=Parallel  TimeDomain=Continuous-time  UseExternalTs=off  SampleTime=-1  IntegratorMethod=Forward Euler  FilterMethod=Forward Euler  ControllerParametersSource=internal  P=160  I=30  UseKiTs=off  D=150  N=1000  UseFilter=on  TunerSelectOption=Transfer Function Based (PID Tuner App)  InitialConditionSource=internal  InitialConditionForIntegrator=0  InitialConditionForFilter=0  DifferentiatorICPrevScaledInput=0  ExternalReset=none  TrackingMode=off  Kt=1  LimitOutput=off  SatLimitsSource=internal  UpperSaturationLimit=inf  LowerSaturationLimit=-inf  LinearizeAsGain=on  AntiWindupMode=none  Kb=1  POutMin=[]  POutMax=[]  IOutMin=[]  IOutMax=[]  DOutMin=[]  DOutMax=[]  NOutMin=[]  NOutMax=[]  SumOutMin=[]  SumOutMax=[]  SaturationOutMin=[]  SaturationOutMax=[]  PParamMin=[]  PParamMax=[]  IParamMin=[]  IParamMax=[]  DParamMin=[]  DParamMax=[]  NParamMin=[]  NParamMax=[]  KbParamMin=[]  KbParamMax=[]  KtParamMin=[]  KtParamMax=[]  KbOutMin=[]  KbOutMax=[]  KtOutMin=[]  KtOutMax=[]  IntegratorOutMin=[]  IntegratorOutMax=[]  FilterOutMin=[]  FilterOutMax=[]  SumI1OutMin=[]  SumI1OutMax=[]  SumI2OutMin=[]  SumI2OutMax=[]  SumI3OutMin=[]  SumI3OutMax=[]  SumI4OutMin=[]  SumI4OutMax=[]  SumDOutMin=[]  SumDOutMax=[]  DifferentiatorOutMin=[]  DifferentiatorOutMax=[]  FilterDiffOutCoefMin=[]  FilterDiffOutCoefMax=[]  ReciprocalOutMin=[]  ReciprocalOutMax=[]  SumDenOutMin=[]  SumDenOutMax=[]  SumNumOutMin=[]  SumNumOutMax=[]  DivideOutMin=[]  DivideOutMax=[]  UdiffTsProdOutMin=[]  UdiffTsProdOutMax=[]  NTsProdOutMin=[]  NTsProdOutMax=[]  UintegralTsProdOutMin=[]  UintegralTsProdOutMax=[]  UngainTsProdOutMin=[]  UngainTsProdOutMax=[]  IntegratorContinuousStateAttributes=''  IntegratorStateMustResolveToSignalObject=off  IntegratorRTWStateStorageClass=Auto  FilterContinuousStateAttributes=''  FilterStateMustResolveToSignalObject=off  FilterRTWStateStorageClass=Auto  ParallelPVariant=InternalParameters  IdealPVariant=Disabled  IVariant=InternalParameters  DVariant=InternalParameters  IntegratorVariant=Continuous  SatVariant=Disabled  AWVariant=Passthrough  PCopyVariant=Disabled  TRVariant=Disabled  FdbkBlocksVariant=Forward  IdealPFdbkVariant=Disabled  SatFdbkVariant=Disabled  DerivativeFilterVariant=ContFilter  NVariant=InternalParameters  NCopyVariant=Disabled  FilterICVariant=InternalICsFilter  IntegratorICVariant=InternalICs  ExternalResetVariant=Disabled  TRSumVariant=Passthrough  SumFdbkVariant=Disabled  SumVariant=Sum_PID  TsampFilterVariant=InternalTs  TsampNgainVariant=Passthrough  TsampIntegralVariant=Passthrough  ExternalSaturationOutDataTypeStr=Inherit: Same as second input  aMode=0
  Sum : Sum  Inputs=|+-
  Sum1 : Sum  Inputs=|+-
  Sum2 : Sum  Inputs=|+-
  u2 : Outport
  u3 : Outport  Port=2
  u4 : Outport  Port=3
  wires:
  fan0/1 -> Sum/1
  fan/1 -> Sum/2
  theta0/1 -> Sum1/1
  theta/1 -> Sum1/2
  psi0/1 -> Sum2/1
  psi/1 -> Sum2/2
  Sum/1 -> PID Controller/1
  Sum1/1 -> PID Controller1/1
  Sum2/1 -> PID Controller2/1
  PID Controller/1 -> Gain/1
  Gain/1 -> u2/1
  PID Controller2/1 -> Gain2/1
  PID Controller1/1 -> Gain1/1
  Gain2/1 -> u4/1
  Gain1/1 -> u3/1
